simulink library "system_blocks"  (Simulink 8.4)
settings: Solver=ode45  SolverMode=SingleTasking  StartTime=0.0  StopTime=10.0  RelTol=1e-3
values from neighbouring files (symbols this model uses):
  A = 'STP1'    [digital_communications_gui.m]
  D = 'STP4'    [digital_communications_gui.m]
  T = 273+20    (= 293)    [exercise_00.m]
undefined symbols (not defined in the file or in its folder): T4
libraries: simulink x9, dspswit3 x5, dspsigops x2, dspobslib x2, dsparch4 x1, simulink_extras x1, dspmtrx3 x1
(part 2 of 2)

== system system_blocks/8 bit Parallel-Serial/D Flip-Flop5 ==
  D : Inport
  CLK : Inport  Port=2
  Constant1 : Constant
  D Flip-Flop : Subsystem  TreatAsAtomicUnit=on
  Data Type Conversion : DataTypeConversion  OutDataTypeStr=boolean  SaturateOnIntegerOverflow=on  RndMeth=Zero
  Q : Outport  InitialOutput=0
  !Q : Outport  Port=2  InitialOutput=1
  wires:
  Constant1/1 -> Data Type Conversion/1
  Data Type Conversion/1 -> D Flip-Flop/Enable
  CLK/1 -> D Flip-Flop/Trigger
  D Flip-Flop/1(Q) -> Q/1
  D/1 -> D Flip-Flop/1(D)
  D Flip-Flop/2(!Q) -> !Q/1

== system system_blocks/8 bit Parallel-Serial/D Flip-Flop6 ==
  D : Inport
  CLK : Inport  Port=2
  Constant1 : Constant
  D Flip-Flop : Subsystem  TreatAsAtomicUnit=on
  Data Type Conversion : DataTypeConversion  OutDataTypeStr=boolean  SaturateOnIntegerOverflow=on  RndMeth=Zero
  Q : Outport  InitialOutput=0
  !Q : Outport  Port=2  InitialOutput=1
  wires:
  Constant1/1 -> Data Type Conversion/1
  Data Type Conversion/1 -> D Flip-Flop/Enable
  CLK/1 -> D Flip-Flop/Trigger
  D Flip-Flop/1(Q) -> Q/1
  D/1 -> D Flip-Flop/1(D)
  D Flip-Flop/2(!Q) -> !Q/1

== system system_blocks/8 bit Parallel-Serial/D Flip-Flop7 ==
  D : Inport
  CLK : Inport  Port=2
  Constant1 : Constant
  D Flip-Flop : Subsystem  TreatAsAtomicUnit=on
  Data Type Conversion : DataTypeConversion  OutDataTypeStr=boolean  SaturateOnIntegerOverflow=on  RndMeth=Zero
  Q : Outport  InitialOutput=0
  !Q : Outport  Port=2  InitialOutput=1
  wires:
  Constant1/1 -> Data Type Conversion/1
  Data Type Conversion/1 -> D Flip-Flop/Enable
  CLK/1 -> D Flip-Flop/Trigger
  D Flip-Flop/1(Q) -> Q/1
  D/1 -> D Flip-Flop/1(D)
  D Flip-Flop/2(!Q) -> !Q/1

== system system_blocks/8 bit Parallel-Serial/D Flip-Flop8 ==
  D : Inport
  CLK : Inport  Port=2
  Constant1 : Constant
  D Flip-Flop : Subsystem  TreatAsAtomicUnit=on
  Data Type Conversion : DataTypeConversion  OutDataTypeStr=boolean  SaturateOnIntegerOverflow=on  RndMeth=Zero
  Q : Outport  InitialOutput=0
  !Q : Outport  Port=2  InitialOutput=1
  wires:
  Constant1/1 -> Data Type Conversion/1
  Data Type Conversion/1 -> D Flip-Flop/Enable
  CLK/1 -> D Flip-Flop/Trigger
  D Flip-Flop/1(Q) -> Q/1
  D/1 -> D Flip-Flop/1(D)
  D Flip-Flop/2(!Q) -> !Q/1

== system system_blocks/8 bit Serial-Parallel/D Flip-Flop1 ==
  D : Inport
  CLK : Inport  Port=2
  Constant1 : Constant
  D Flip-Flop : Subsystem  TreatAsAtomicUnit=on
  Data Type Conversion : DataTypeConversion  OutDataTypeStr=boolean  SaturateOnIntegerOverflow=on  RndMeth=Zero
  Q : Outport  InitialOutput=0
  !Q : Outport  Port=2  InitialOutput=1
  wires:
  Constant1/1 -> Data Type Conversion/1
  Data Type Conversion/1 -> D Flip-Flop/Enable
  CLK/1 -> D Flip-Flop/Trigger
  D Flip-Flop/1(Q) -> Q/1
  D/1 -> D Flip-Flop/1(D)
  D Flip-Flop/2(!Q) -> !Q/1

== system system_blocks/8 bit Serial-Parallel/D Flip-Flop10 ==
  D : Inport
  CLK : Inport  Port=2
  Constant1 : Constant
  D Flip-Flop : Subsystem  TreatAsAtomicUnit=on
  Data Type Conversion : DataTypeConversion  OutDataTypeStr=boolean  SaturateOnIntegerOverflow=on  RndMeth=Zero
  Q : Outport  InitialOutput=0
  wires:
  Constant1/1 -> Data Type Conversion/1
  Data Type Conversion/1 -> D Flip-Flop/Enable
  CLK/1 -> D Flip-Flop/Trigger
  D Flip-Flop/1(Q) -> Q/1
  D/1 -> D Flip-Flop/1(D)

== system system_blocks/8 bit Serial-Parallel/D Flip-Flop11 ==
  D : Inport
  CLK : Inport  Port=2
  Constant1 : Constant
  D Flip-Flop : Subsystem  TreatAsAtomicUnit=on
  Data Type Conversion : DataTypeConversion  OutDataTypeStr=boolean  SaturateOnIntegerOverflow=on  RndMeth=Zero
  Q : Outport  InitialOutput=0
  wires:
  Constant1/1 -> Data Type Conversion/1
  Data Type Conversion/1 -> D Flip-Flop/Enable
  CLK/1 -> D Flip-Flop/Trigger
  D Flip-Flop/1(Q) -> Q/1
  D/1 -> D Flip-Flop/1(D)

== system system_blocks/8 bit Serial-Parallel/D Flip-Flop12 ==
  D : Inport
  CLK : Inport  Port=2
  Constant1 : Constant
  D Flip-Flop : Subsystem  TreatAsAtomicUnit=on
  Data Type Conversion : DataTypeConversion  OutDataTypeStr=boolean  SaturateOnIntegerOverflow=on  RndMeth=Zero
  Q : Outport  InitialOutput=0
  wires:
  Constant1/1 -> Data Type Conversion/1
  Data Type Conversion/1 -> D Flip-Flop/Enable
  CLK/1 -> D Flip-Flop/Trigger
  D Flip-Flop/1(Q) -> Q/1
  D/1 -> D Flip-Flop/1(D)

== system system_blocks/8 bit Serial-Parallel/D Flip-Flop13 ==
  D : Inport
  CLK : Inport  Port=2
  Constant1 : Constant
  D Flip-Flop : Subsystem  TreatAsAtomicUnit=on
  Data Type Conversion : DataTypeConversion  OutDataTypeStr=boolean  SaturateOnIntegerOverflow=on  RndMeth=Zero
  Q : Outport  InitialOutput=0
  wires:
  Constant1/1 -> Data Type Conversion/1
  Data Type Conversion/1 -> D Flip-Flop/Enable
  CLK/1 -> D Flip-Flop/Trigger
  D Flip-Flop/1(Q) -> Q/1
  D/1 -> D Flip-Flop/1(D)

== system system_blocks/8 bit Serial-Parallel/D Flip-Flop14 ==
  D : Inport
  CLK : Inport  Port=2
  Constant1 : Constant
  D Flip-Flop : Subsystem  TreatAsAtomicUnit=on
  Data Type Conversion : DataTypeConversion  OutDataTypeStr=boolean  SaturateOnIntegerOverflow=on  RndMeth=Zero
  Q : Outport  InitialOutput=0
  wires:
  Constant1/1 -> Data Type Conversion/1
  Data Type Conversion/1 -> D Flip-Flop/Enable
  CLK/1 -> D Flip-Flop/Trigger
  D Flip-Flop/1(Q) -> Q/1
  D/1 -> D Flip-Flop/1(D)

== system system_blocks/8 bit Serial-Parallel/D Flip-Flop15 ==
  D : Inport
  CLK : Inport  Port=2
  Constant1 : Constant
  D Flip-Flop : Subsystem  TreatAsAtomicUnit=on
  Data Type Conversion : DataTypeConversion  OutDataTypeStr=boolean  SaturateOnIntegerOverflow=on  RndMeth=Zero
  Q : Outport  InitialOutput=0
  wires:
  Constant1/1 -> Data Type Conversion/1
  Data Type Conversion/1 -> D Flip-Flop/Enable
  CLK/1 -> D Flip-Flop/Trigger
  D Flip-Flop/1(Q) -> Q/1
  D/1 -> D Flip-Flop/1(D)

== system system_blocks/8 bit Serial-Parallel/D Flip-Flop16 ==
  D : Inport
  CLK : Inport  Port=2
  Constant1 : Constant
  D Flip-Flop : Subsystem  TreatAsAtomicUnit=on
  Data Type Conversion : DataTypeConversion  OutDataTypeStr=boolean  SaturateOnIntegerOverflow=on  RndMeth=Zero
  Q : Outport  InitialOutput=0
  wires:
  Constant1/1 -> Data Type Conversion/1
  Data Type Conversion/1 -> D Flip-Flop/Enable
  CLK/1 -> D Flip-Flop/Trigger
  D Flip-Flop/1(Q) -> Q/1
  D/1 -> D Flip-Flop/1(D)

== system system_blocks/8 bit Serial-Parallel/D Flip-Flop2 ==
  D : Inport
  CLK : Inport  Port=2
  Constant1 : Constant
  D Flip-Flop : Subsystem  TreatAsAtomicUnit=on
  Data Type Conversion : DataTypeConversion  OutDataTypeStr=boolean  SaturateOnIntegerOverflow=on  RndMeth=Zero
  Q : Outport  InitialOutput=0
  !Q : Outport  Port=2  InitialOutput=1
  wires:
  Constant1/1 -> Data Type Conversion/1
  Data Type Conversion/1 -> D Flip-Flop/Enable
  CLK/1 -> D Flip-Flop/Trigger
  D Flip-Flop/1(Q) -> Q/1
  D/1 -> D Flip-Flop/1(D)
  D Flip-Flop/2(!Q) -> !Q/1

== system system_blocks/8 bit Serial-Parallel/D Flip-Flop3 ==
  D : Inport
  CLK : Inport  Port=2
  Constant1 : Constant
  D Flip-Flop : Subsystem  TreatAsAtomicUnit=on
  Data Type Conversion : DataTypeConversion  OutDataTypeStr=boolean  SaturateOnIntegerOverflow=on  RndMeth=Zero
  Q : Outport  InitialOutput=0
  !Q : Outport  Port=2  InitialOutput=1
  wires:
  Constant1/1 -> Data Type Conversion/1
  Data Type Conversion/1 -> D Flip-Flop/Enable
  CLK/1 -> D Flip-Flop/Trigger
  D Flip-Flop/1(Q) -> Q/1
  D/1 -> D Flip-Flop/1(D)
  D Flip-Flop/2(!Q) -> !Q/1

== system system_blocks/8 bit Serial-Parallel/D Flip-Flop4 ==
  D : Inport
  CLK : Inport  Port=2
  Constant1 : Constant
  D Flip-Flop : Subsystem  TreatAsAtomicUnit=on
  Data Type Conversion : DataTypeConversion  OutDataTypeStr=boolean  SaturateOnIntegerOverflow=on  RndMeth=Zero
  Q : Outport  InitialOutput=0
  !Q : Outport  Port=2  InitialOutput=1
  wires:
  Constant1/1 -> Data Type Conversion/1
  Data Type Conversion/1 -> D Flip-Flop/Enable
  CLK/1 -> D Flip-Flop/Trigger
  D Flip-Flop/1(Q) -> Q/1
  D/1 -> D Flip-Flop/1(D)
  D Flip-Flop/2(!Q) -> !Q/1

== system system_blocks/8 bit Serial-Parallel/D Flip-Flop5 ==
  D : Inport
  CLK : Inport  Port=2
  Constant1 : Constant
  D Flip-Flop : Subsystem  TreatAsAtomicUnit=on
  Data Type Conversion : DataTypeConversion  OutDataTypeStr=boolean  SaturateOnIntegerOverflow=on  RndMeth=Zero
  Q : Outport  InitialOutput=0
  !Q : Outport  Port=2  InitialOutput=1
  wires:
  Constant1/1 -> Data Type Conversion/1
  Data Type Conversion/1 -> D Flip-Flop/Enable
  CLK/1 -> D Flip-Flop/Trigger
  D Flip-Flop/1(Q) -> Q/1
  D/1 -> D Flip-Flop/1(D)
  D Flip-Flop/2(!Q) -> !Q/1

== system system_blocks/8 bit Serial-Parallel/D Flip-Flop6 ==
  D : Inport
  CLK : Inport  Port=2
  Constant1 : Constant
  D Flip-Flop : Subsystem  TreatAsAtomicUnit=on
  Data Type Conversion : DataTypeConversion  OutDataTypeStr=boolean  SaturateOnIntegerOverflow=on  RndMeth=Zero
  Q : Outport  InitialOutput=0
  !Q : Outport  Port=2  InitialOutput=1
  wires:
  Constant1/1 -> Data Type Conversion/1
  Data Type Conversion/1 -> D Flip-Flop/Enable
  CLK/1 -> D Flip-Flop/Trigger
  D Flip-Flop/1(Q) -> Q/1
  D/1 -> D Flip-Flop/1(D)
  D Flip-Flop/2(!Q) -> !Q/1

== system system_blocks/8 bit Serial-Parallel/D Flip-Flop7 ==
  D : Inport
  CLK : Inport  Port=2
  Constant1 : Constant
  D Flip-Flop : Subsystem  TreatAsAtomicUnit=on
  Data Type Conversion : DataTypeConversion  OutDataTypeStr=boolean  SaturateOnIntegerOverflow=on  RndMeth=Zero
  Q : Outport  InitialOutput=0
  !Q : Outport  Port=2  InitialOutput=1
  wires:
  Constant1/1 -> Data Type Conversion/1
  Data Type Conversion/1 -> D Flip-Flop/Enable
  CLK/1 -> D Flip-Flop/Trigger
  D Flip-Flop/1(Q) -> Q/1
  D/1 -> D Flip-Flop/1(D)
  D Flip-Flop/2(!Q) -> !Q/1

== system system_blocks/8 bit Serial-Parallel/D Flip-Flop8 ==
  D : Inport
  CLK : Inport  Port=2
  Constant1 : Constant
  D Flip-Flop : Subsystem  TreatAsAtomicUnit=on
  Data Type Conversion : DataTypeConversion  OutDataTypeStr=boolean  SaturateOnIntegerOverflow=on  RndMeth=Zero
  Q : Outport  InitialOutput=0
  !Q : Outport  Port=2  InitialOutput=1
  wires:
  Constant1/1 -> Data Type Conversion/1
  Data Type Conversion/1 -> D Flip-Flop/Enable
  CLK/1 -> D Flip-Flop/Trigger
  D Flip-Flop/1(Q) -> Q/1
  D/1 -> D Flip-Flop/1(D)
  D Flip-Flop/2(!Q) -> !Q/1

== system system_blocks/8 bit Serial-Parallel/D Flip-Flop9 ==
  D : Inport
  CLK : Inport  Port=2
  Constant1 : Constant
  D Flip-Flop : Subsystem  TreatAsAtomicUnit=on
  Data Type Conversion : DataTypeConversion  OutDataTypeStr=boolean  SaturateOnIntegerOverflow=on  RndMeth=Zero
  Q : Outport  InitialOutput=0
  wires:
  Constant1/1 -> Data Type Conversion/1
  Data Type Conversion/1 -> D Flip-Flop/Enable
  CLK/1 -> D Flip-Flop/Trigger
  D Flip-Flop/1(Q) -> Q/1
  D/1 -> D Flip-Flop/1(D)

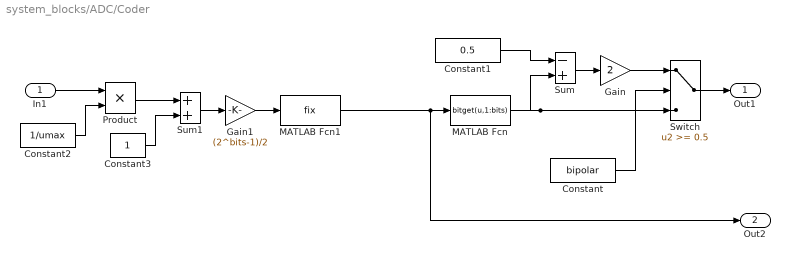
== system system_blocks/ADC/Coder ==
  In1 : Inport
  Constant : Constant  Value=bipolar
  Constant1 : Constant  Value=0.5
  Constant2 : Constant  Value=1/umax
  Constant3 : Constant
  Gain : Gain  Gain=2  SaturateOnIntegerOverflow=on  OutDataTypeStr=Inherit: Same as input  ParamDataTypeStr=Inherit: Same as input
  Gain1 : Gain  Gain=(2^bits-1)/2  SaturateOnIntegerOverflow=on  OutDataTypeStr=Inherit: Same as input  ParamDataTypeStr=Inherit: Same as input
  MATLAB Fcn : MATLABFcn  MATLABFcn=bitget(u,1:bits)  OutputDimensions=bits
  MATLAB Fcn1 : MATLABFcn  MATLABFcn=fix  OutputDimensions=1
  Product : Product  SaturateOnIntegerOverflow=on  InputSameDT=on  OutDataTypeStr=Inherit: Same as first input
  Sum : Sum  Inputs=-+  SaturateOnIntegerOverflow=on  InputSameDT=on  OutDataTypeStr=Inherit: Same as first input
  Sum1 : Sum  SaturateOnIntegerOverflow=on  InputSameDT=on  OutDataTypeStr=Inherit: Same as first input
  Switch : Switch  Threshold=0.5  SaturateOnIntegerOverflow=on  InputSameDT=on
  Out1 : Outport
  Out2 : Outport  Port=2
  wires:
  Gain1/1 -> MATLAB Fcn1/1
  Sum1/1 -> Gain1/1
  Constant3/1 -> Sum1/2
  Product/1 -> Sum1/1
  Constant2/1 -> Product/2
  In1/1 -> Product/1
  MATLAB Fcn1/1 -> Out2/1, MATLAB Fcn/1
  Constant/1 -> Switch/2
  Gain/1 -> Switch/1
  Sum/1 -> Gain/1
  Constant1/1 -> Sum/1
  MATLAB Fcn/1 -> Sum/2, Switch/3
  Switch/1 -> Out1/1

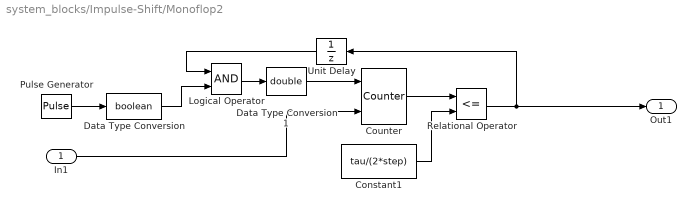
== system system_blocks/Impulse-Shift/Monoflop2 ==
  In1 : Inport
  Constant1 : Constant  Value=tau/(2*step)
  Counter : dspswit3/Counter  Direction=Up  CountEvent=Rising edge  CounterSize=User defined  MaxCount=ceil(tau/(2*step))+1  InitialCount=0  Output=Count  HitValue=1  ResetInput=on  SamplesPerFrame=1  Ts=1  CntDtype=double  HitDtype=Boolean
  Data Type Conversion : DataTypeConversion  OutDataTypeStr=boolean  SaturateOnIntegerOverflow=on  RndMeth=Zero
  Data Type Conversion1 : DataTypeConversion  OutDataTypeStr=double  SaturateOnIntegerOverflow=on  RndMeth=Zero
  Logical Operator : Logic  AllPortsSameDT=off
  Pulse Generator : DiscretePulseGenerator  PulseType=Time based  Period=2*step  PulseWidth=50
  Relational Operator : RelationalOperator  Operator=<=
  Unit Delay : UnitDelay  SampleTime=step
  Out1 : Outport
  wires:
  Unit Delay/1 -> Logical Operator/1
  In1/1 -> Counter/2
  Data Type Conversion1/1 -> Counter/1
  Logical Operator/1 -> Data Type Conversion1/1
  Data Type Conversion/1 -> Logical Operator/2
  Pulse Generator/1 -> Data Type Conversion/1
  Relational Operator/1 -> Unit Delay/1, Out1/1
  Constant1/1 -> Relational Operator/2
  Counter/1 -> Relational Operator/1

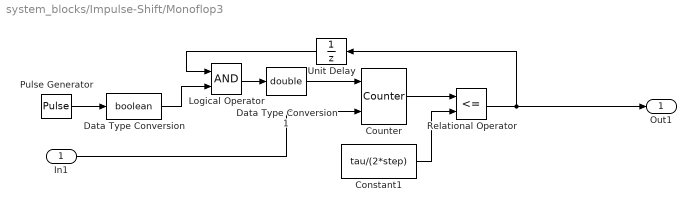
== system system_blocks/Impulse-Shift/Monoflop3 ==
  In1 : Inport
  Constant1 : Constant  Value=tau/(2*step)
  Counter : dspswit3/Counter  Direction=Up  CountEvent=Rising edge  CounterSize=User defined  MaxCount=ceil(tau/(2*step))+1  InitialCount=0  Output=Count  HitValue=1  ResetInput=on  SamplesPerFrame=1  Ts=1  CntDtype=double  HitDtype=Boolean
  Data Type Conversion : DataTypeConversion  OutDataTypeStr=boolean  SaturateOnIntegerOverflow=on  RndMeth=Zero
  Data Type Conversion1 : DataTypeConversion  OutDataTypeStr=double  SaturateOnIntegerOverflow=on  RndMeth=Zero
  Logical Operator : Logic  AllPortsSameDT=off
  Pulse Generator : DiscretePulseGenerator  PulseType=Time based  Period=2*step  PulseWidth=50
  Relational Operator : RelationalOperator  Operator=<=
  Unit Delay : UnitDelay  SampleTime=step
  Out1 : Outport
  wires:
  Unit Delay/1 -> Logical Operator/1
  In1/1 -> Counter/2
  Data Type Conversion1/1 -> Counter/1
  Logical Operator/1 -> Data Type Conversion1/1
  Data Type Conversion/1 -> Logical Operator/2
  Pulse Generator/1 -> Data Type Conversion/1
  Relational Operator/1 -> Unit Delay/1, Out1/1
  Constant1/1 -> Relational Operator/2
  Counter/1 -> Relational Operator/1

== system system_blocks/Repeater/Clock Recovery ==
  In : Inport
  Formatwandlung : Subsystem
  Loop Filter : Subsystem  mask{Typ=Typ}
      mask prompts: Typ "Schleifenfilter"
      mask init:
      | T3=1e-5, T4=T3
      | 
      | if Typ==1,
      | 	T1=8.2e-3
      | 	T2=1.804e-3
      | 	
      | elseif Typ==2,
      | 	T1=2.2e-3
      | 	T2=1.32e-3
      | 	
      | else T1=0.82e-3;
      | 	 T2=1.23e-3;
      | 	 
      |  end
  Phasen- diskriminator : Subsystem
  VCO : Subsystem  mask{fo=fbit, Typ=Typ}
      mask prompts: fo "Ruhefrequenz"; Typ "Schleifenfilter"
      mask init:
      | if Typ == 1,
      | 	Ki = 9972
      | 	
      | elseif Typ == 2,
      | 		Ki = 5569
      | 		
      | 	else Ki= 2926
      | 		
      | end
  clock signal : Outport
  VCO_sin : Outport  Port=2
  wires:
  VCO/2(VCO_sin) -> VCO_sin/1
  VCO/1(VCO_rect) -> clock signal/1, Phasen- diskriminator/2(VCO_rect)
  Loop Filter/1(Out1) -> VCO/1(In1)
  Phasen- diskriminator/1(Out) -> Loop Filter/1(In1)
  Formatwandlung/1(Out1) -> Phasen- diskriminator/1(Data)
  In/1 -> Formatwandlung/1(In1)

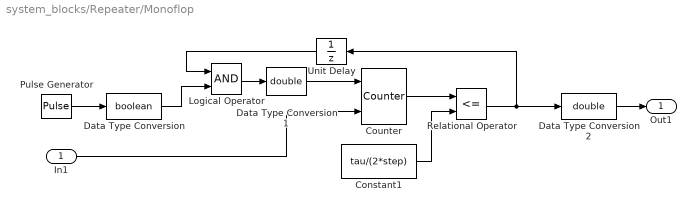
== system system_blocks/Repeater/Monoflop ==
  In1 : Inport
  Constant1 : Constant  Value=tau/(2*step)
  Counter : dspswit3/Counter  Direction=Up  CountEvent=Rising edge  CounterSize=User defined  MaxCount=ceil(tau/(2*step))+1  InitialCount=0  Output=Count  HitValue=1  ResetInput=on  SamplesPerFrame=1  Ts=1  CntDtype=double  HitDtype=Boolean
  Data Type Conversion : DataTypeConversion  OutDataTypeStr=boolean  SaturateOnIntegerOverflow=on  RndMeth=Zero
  Data Type Conversion1 : DataTypeConversion  OutDataTypeStr=double  SaturateOnIntegerOverflow=on  RndMeth=Zero
  Data Type Conversion2 : DataTypeConversion  OutDataTypeStr=double  SaturateOnIntegerOverflow=on  RndMeth=Zero
  Logical Operator : Logic  AllPortsSameDT=off
  Pulse Generator : DiscretePulseGenerator  PulseType=Time based  Period=2*step  PulseWidth=50
  Relational Operator : RelationalOperator  Operator=<=
  Unit Delay : UnitDelay  SampleTime=step
  Out1 : Outport
  wires:
  Data Type Conversion2/1 -> Out1/1
  Unit Delay/1 -> Logical Operator/1
  In1/1 -> Counter/2
  Data Type Conversion1/1 -> Counter/1
  Logical Operator/1 -> Data Type Conversion1/1
  Data Type Conversion/1 -> Logical Operator/2
  Pulse Generator/1 -> Data Type Conversion/1
  Relational Operator/1 -> Data Type Conversion2/1, Unit Delay/1
  Constant1/1 -> Relational Operator/2
  Counter/1 -> Relational Operator/1

== system system_blocks/8 bit Parallel-Serial/D Flip-Flop1/D Flip-Flop ==
  D : Inport  LatchByDelayingOutsideSignal=on
  C : EnablePort
  Trigger : TriggerPort
  Logic : Logic  Operator=NOT  Inputs=1
  Q : Outport  OutputWhenDisabled=reset  InitialOutput=0
  !Q : Outport  Port=2  OutputWhenDisabled=reset  InitialOutput=1
  wires:
  Logic/1 -> !Q/1
  D/1 -> Q/1, Logic/1

== system system_blocks/8 bit Parallel-Serial/D Flip-Flop2/D Flip-Flop ==
  D : Inport  LatchByDelayingOutsideSignal=on
  C : EnablePort
  Trigger : TriggerPort
  Logic : Logic  Operator=NOT  Inputs=1
  Q : Outport  OutputWhenDisabled=reset  InitialOutput=0
  !Q : Outport  Port=2  OutputWhenDisabled=reset  InitialOutput=1
  wires:
  Logic/1 -> !Q/1
  D/1 -> Q/1, Logic/1

== system system_blocks/8 bit Parallel-Serial/D Flip-Flop3/D Flip-Flop ==
  D : Inport  LatchByDelayingOutsideSignal=on
  C : EnablePort
  Trigger : TriggerPort
  Logic : Logic  Operator=NOT  Inputs=1
  Q : Outport  OutputWhenDisabled=reset  InitialOutput=0
  !Q : Outport  Port=2  OutputWhenDisabled=reset  InitialOutput=1
  wires:
  Logic/1 -> !Q/1
  D/1 -> Q/1, Logic/1

== system system_blocks/8 bit Parallel-Serial/D Flip-Flop4/D Flip-Flop ==
  D : Inport  LatchByDelayingOutsideSignal=on
  C : EnablePort
  Trigger : TriggerPort
  Logic : Logic  Operator=NOT  Inputs=1
  Q : Outport  OutputWhenDisabled=reset  InitialOutput=0
  !Q : Outport  Port=2  OutputWhenDisabled=reset  InitialOutput=1
  wires:
  Logic/1 -> !Q/1
  D/1 -> Q/1, Logic/1

== system system_blocks/8 bit Parallel-Serial/D Flip-Flop5/D Flip-Flop ==
  D : Inport  LatchByDelayingOutsideSignal=on
  C : EnablePort
  Trigger : TriggerPort
  Logic : Logic  Operator=NOT  Inputs=1
  Q : Outport  OutputWhenDisabled=reset  InitialOutput=0
  !Q : Outport  Port=2  OutputWhenDisabled=reset  InitialOutput=1
  wires:
  Logic/1 -> !Q/1
  D/1 -> Q/1, Logic/1

== system system_blocks/8 bit Parallel-Serial/D Flip-Flop6/D Flip-Flop ==
  D : Inport  LatchByDelayingOutsideSignal=on
  C : EnablePort
  Trigger : TriggerPort
  Logic : Logic  Operator=NOT  Inputs=1
  Q : Outport  OutputWhenDisabled=reset  InitialOutput=0
  !Q : Outport  Port=2  OutputWhenDisabled=reset  InitialOutput=1
  wires:
  Logic/1 -> !Q/1
  D/1 -> Q/1, Logic/1

== system system_blocks/8 bit Parallel-Serial/D Flip-Flop7/D Flip-Flop ==
  D : Inport  LatchByDelayingOutsideSignal=on
  C : EnablePort
  Trigger : TriggerPort
  Logic : Logic  Operator=NOT  Inputs=1
  Q : Outport  OutputWhenDisabled=reset  InitialOutput=0
  !Q : Outport  Port=2  OutputWhenDisabled=reset  InitialOutput=1
  wires:
  Logic/1 -> !Q/1
  D/1 -> Q/1, Logic/1

== system system_blocks/8 bit Parallel-Serial/D Flip-Flop8/D Flip-Flop ==
  D : Inport  LatchByDelayingOutsideSignal=on
  C : EnablePort
  Trigger : TriggerPort
  Logic : Logic  Operator=NOT  Inputs=1
  Q : Outport  OutputWhenDisabled=reset  InitialOutput=0
  !Q : Outport  Port=2  OutputWhenDisabled=reset  InitialOutput=1
  wires:
  Logic/1 -> !Q/1
  D/1 -> Q/1, Logic/1

== system system_blocks/8 bit Serial-Parallel/D Flip-Flop1/D Flip-Flop ==
  D : Inport  LatchByDelayingOutsideSignal=on
  C : EnablePort
  Trigger : TriggerPort
  Logic : Logic  Operator=NOT  Inputs=1
  Q : Outport  OutputWhenDisabled=reset  InitialOutput=0
  !Q : Outport  Port=2  OutputWhenDisabled=reset  InitialOutput=1
  wires:
  Logic/1 -> !Q/1
  D/1 -> Q/1, Logic/1

== system system_blocks/8 bit Serial-Parallel/D Flip-Flop10/D Flip-Flop ==
  D : Inport  LatchByDelayingOutsideSignal=on
  C : EnablePort
  Trigger : TriggerPort
  Q : Outport  OutputWhenDisabled=reset  InitialOutput=0
  wires:
  D/1 -> Q/1

== system system_blocks/8 bit Serial-Parallel/D Flip-Flop11/D Flip-Flop ==
  D : Inport  LatchByDelayingOutsideSignal=on
  C : EnablePort
  Trigger : TriggerPort
  Q : Outport  OutputWhenDisabled=reset  InitialOutput=0
  wires:
  D/1 -> Q/1

== system system_blocks/8 bit Serial-Parallel/D Flip-Flop12/D Flip-Flop ==
  D : Inport  LatchByDelayingOutsideSignal=on
  C : EnablePort
  Trigger : TriggerPort
  Q : Outport  OutputWhenDisabled=reset  InitialOutput=0
  wires:
  D/1 -> Q/1

== system system_blocks/8 bit Serial-Parallel/D Flip-Flop13/D Flip-Flop ==
  D : Inport  LatchByDelayingOutsideSignal=on
  C : EnablePort
  Trigger : TriggerPort
  Q : Outport  OutputWhenDisabled=reset  InitialOutput=0
  wires:
  D/1 -> Q/1

== system system_blocks/8 bit Serial-Parallel/D Flip-Flop14/D Flip-Flop ==
  D : Inport  LatchByDelayingOutsideSignal=on
  C : EnablePort
  Trigger : TriggerPort
  Q : Outport  OutputWhenDisabled=reset  InitialOutput=0
  wires:
  D/1 -> Q/1

== system system_blocks/8 bit Serial-Parallel/D Flip-Flop15/D Flip-Flop ==
  D : Inport  LatchByDelayingOutsideSignal=on
  C : EnablePort
  Trigger : TriggerPort
  Q : Outport  OutputWhenDisabled=reset  InitialOutput=0
  wires:
  D/1 -> Q/1

== system system_blocks/8 bit Serial-Parallel/D Flip-Flop16/D Flip-Flop ==
  D : Inport  LatchByDelayingOutsideSignal=on
  C : EnablePort
  Trigger : TriggerPort
  Q : Outport  OutputWhenDisabled=reset  InitialOutput=0
  wires:
  D/1 -> Q/1

== system system_blocks/8 bit Serial-Parallel/D Flip-Flop2/D Flip-Flop ==
  D : Inport  LatchByDelayingOutsideSignal=on
  C : EnablePort
  Trigger : TriggerPort
  Logic : Logic  Operator=NOT  Inputs=1
  Q : Outport  OutputWhenDisabled=reset  InitialOutput=0
  !Q : Outport  Port=2  OutputWhenDisabled=reset  InitialOutput=1
  wires:
  Logic/1 -> !Q/1
  D/1 -> Q/1, Logic/1

== system system_blocks/8 bit Serial-Parallel/D Flip-Flop3/D Flip-Flop ==
  D : Inport  LatchByDelayingOutsideSignal=on
  C : EnablePort
  Trigger : TriggerPort
  Logic : Logic  Operator=NOT  Inputs=1
  Q : Outport  OutputWhenDisabled=reset  InitialOutput=0
  !Q : Outport  Port=2  OutputWhenDisabled=reset  InitialOutput=1
  wires:
  Logic/1 -> !Q/1
  D/1 -> Q/1, Logic/1

== system system_blocks/8 bit Serial-Parallel/D Flip-Flop4/D Flip-Flop ==
  D : Inport  LatchByDelayingOutsideSignal=on
  C : EnablePort
  Trigger : TriggerPort
  Logic : Logic  Operator=NOT  Inputs=1
  Q : Outport  OutputWhenDisabled=reset  InitialOutput=0
  !Q : Outport  Port=2  OutputWhenDisabled=reset  InitialOutput=1
  wires:
  Logic/1 -> !Q/1
  D/1 -> Q/1, Logic/1

== system system_blocks/8 bit Serial-Parallel/D Flip-Flop5/D Flip-Flop ==
  D : Inport  LatchByDelayingOutsideSignal=on
  C : EnablePort
  Trigger : TriggerPort
  Logic : Logic  Operator=NOT  Inputs=1
  Q : Outport  OutputWhenDisabled=reset  InitialOutput=0
  !Q : Outport  Port=2  OutputWhenDisabled=reset  InitialOutput=1
  wires:
  Logic/1 -> !Q/1
  D/1 -> Q/1, Logic/1

== system system_blocks/8 bit Serial-Parallel/D Flip-Flop6/D Flip-Flop ==
  D : Inport  LatchByDelayingOutsideSignal=on
  C : EnablePort
  Trigger : TriggerPort
  Logic : Logic  Operator=NOT  Inputs=1
  Q : Outport  OutputWhenDisabled=reset  InitialOutput=0
  !Q : Outport  Port=2  OutputWhenDisabled=reset  InitialOutput=1
  wires:
  Logic/1 -> !Q/1
  D/1 -> Q/1, Logic/1

== system system_blocks/8 bit Serial-Parallel/D Flip-Flop7/D Flip-Flop ==
  D : Inport  LatchByDelayingOutsideSignal=on
  C : EnablePort
  Trigger : TriggerPort
  Logic : Logic  Operator=NOT  Inputs=1
  Q : Outport  OutputWhenDisabled=reset  InitialOutput=0
  !Q : Outport  Port=2  OutputWhenDisabled=reset  InitialOutput=1
  wires:
  Logic/1 -> !Q/1
  D/1 -> Q/1, Logic/1

== system system_blocks/8 bit Serial-Parallel/D Flip-Flop8/D Flip-Flop ==
  D : Inport  LatchByDelayingOutsideSignal=on
  C : EnablePort
  Trigger : TriggerPort
  Logic : Logic  Operator=NOT  Inputs=1
  Q : Outport  OutputWhenDisabled=reset  InitialOutput=0
  !Q : Outport  Port=2  OutputWhenDisabled=reset  InitialOutput=1
  wires:
  Logic/1 -> !Q/1
  D/1 -> Q/1, Logic/1

== system system_blocks/8 bit Serial-Parallel/D Flip-Flop9/D Flip-Flop ==
  D : Inport  LatchByDelayingOutsideSignal=on
  C : EnablePort
  Trigger : TriggerPort
  Q : Outport  OutputWhenDisabled=reset  InitialOutput=0
  wires:
  D/1 -> Q/1

== system system_blocks/Repeater/Clock Recovery/Formatwandlung ==
  In1 : Inport
  Abs : Abs  SaturateOnIntegerOverflow=on
  Data Type Conversion : DataTypeConversion  OutDataTypeStr=double  SaturateOnIntegerOverflow=on  RndMeth=Zero
  Data Type Conversion1 : DataTypeConversion  OutDataTypeStr=boolean  SaturateOnIntegerOverflow=on  RndMeth=Zero
  Data Type Conversion2 : DataTypeConversion  OutDataTypeStr=boolean  SaturateOnIntegerOverflow=on  RndMeth=Zero
  Logical Operator : Logic  Operator=XOR
  Relay : Relay  OnSwitchValue=.5  OffSwitchValue=.5
  Transport Delay : TransportDelay  DelayTime=1/(10*fbit)
  Out1 : Outport
  wires:
  Abs/1 -> Relay/1
  Data Type Conversion/1 -> Out1/1
  In1/1 -> Abs/1
  Logical Operator/1 -> Data Type Conversion/1
  Data Type Conversion2/1 -> Logical Operator/2
  Data Type Conversion1/1 -> Logical Operator/1
  Relay/1 -> Data Type Conversion1/1, Transport Delay/1
  Transport Delay/1 -> Data Type Conversion2/1

== system system_blocks/Repeater/Clock Recovery/Loop Filter ==
  In1 : Inport
  Schleifenfilter : TransferFcn  Numerator=[T2 1]  Denominator="[(T4*T3*(T1+T2))  (2*T3*(T1+T2)+T4*(T3-T2+2*(T1+T2)))  (2*(T3-T2)+3*(T1+T2)+T4)  1]"
  Out1 : Outport
  wires:
  Schleifenfilter/1 -> Out1/1
  In1/1 -> Schleifenfilter/1

== system system_blocks/Repeater/Clock Recovery/Phasen- diskriminator ==
  Data : Inport
  VCO_rect : Inport  Port=2
  Constant : Constant  Value=0.5
  Data Type Conversion : DataTypeConversion  OutDataTypeStr=double  SaturateOnIntegerOverflow=on  RndMeth=Zero
  Data Type Conversion1 : DataTypeConversion  OutDataTypeStr=boolean  SaturateOnIntegerOverflow=on  RndMeth=Zero
  Data Type Conversion2 : DataTypeConversion  OutDataTypeStr=boolean  SaturateOnIntegerOverflow=on  RndMeth=Zero
  Gain : Gain  Gain=5  SaturateOnIntegerOverflow=on  OutDataTypeStr=Inherit: Same as input  ParamDataTypeStr=Inherit: Same as input
  Logical Operator : Logic  Operator=XOR
  Sum : Sum  Inputs=+-  SaturateOnIntegerOverflow=on
  Out : Outport
  wires:
  VCO_rect/1 -> Data Type Conversion2/1
  Gain/1 -> Out/1
  Data/1 -> Data Type Conversion1/1
  Sum/1 -> Gain/1
  Constant/1 -> Sum/2
  Data Type Conversion/1 -> Sum/1
  Logical Operator/1 -> Data Type Conversion/1
  Data Type Conversion2/1 -> Logical Operator/2
  Data Type Conversion1/1 -> Logical Operator/1

== system system_blocks/Repeater/Clock Recovery/VCO ==
  In1 : Inport
  Constant1 : Constant  Value=fbit
  Gain : Gain  Gain=Ki/(2*pi)  SaturateOnIntegerOverflow=on  OutDataTypeStr=Inherit: Same as input  ParamDataTypeStr=Inherit: Same as input
  Gain1 : Gain  Gain=2*pi  SaturateOnIntegerOverflow=on  OutDataTypeStr=Inherit: Same as input  ParamDataTypeStr=Inherit: Same as input
  Integrator : Integrator
  Relay : Relay  OffSwitchValue=-eps
  Sum : Sum  SaturateOnIntegerOverflow=on
  Trigonometric Function : Trigonometry
  VCO_rect : Outport
  VCO_sin : Outport  Port=2
  wires:
  Relay/1 -> VCO_rect/1
  In1/1 -> Gain/1
  Trigonometric Function/1 -> VCO_sin/1, Relay/1
  Gain1/1 -> Trigonometric Function/1
  Integrator/1 -> Gain1/1
  Sum/1 -> Integrator/1
  Constant1/1 -> Sum/2
  Gain/1 -> Sum/1
